simulink model "fig529a"  (Simulink 3.00)
settings: Solver=ode45  SolverMode=SingleTasking  StartTime=0.0  StopTime=2  RelTol=1e-3  AbsTol=1e-6
libraries: simulink3 x2

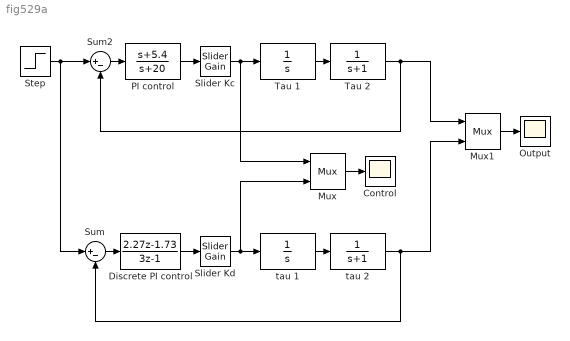
== system fig529a ==
  Control : Scope
      settings: TickLabels=on  TimeRange=auto  YMin=0  YMax=2.75  SaveName=ucd  DataFormat=Matrix
  Discrete PI control : DiscreteTransferFcn  Numerator=[2.27 -1.73]  Denominator=[3 -1]  SampleTime=.05
  Mux : Mux  Inputs=2
      settings: DisplayOption=none
  Mux1 : Mux  Inputs=2
      settings: DisplayOption=none
  Output : Scope
      settings: TickLabels=on  TimeRange=auto  YMin=-5  YMax=5  SaveName=ycd  DataFormat=Matrix
  PI control : TransferFcn  Numerator=[1 5.4]  Denominator=[1 20]
  Slider Kc : simulink3/Math/Slider Gain  low=0  gain=127  high=200
  Slider Kd : simulink3/Math/Slider Gain  low=0  gain=127  high=200
  Step : Step  Time=.1  Before=0  After=1  SampleTime=.001
  Sum : Sum  Inputs=|+-  SaturateOnIntegerOverflow=off
  Sum2 : Sum  Inputs=|+-  SaturateOnIntegerOverflow=off
  Tau 1 : TransferFcn  Numerator=[1]  Denominator=[1 0]
  Tau 2 : TransferFcn  Numerator=[1]  Denominator=[1 1]
  tau 1 : TransferFcn  Numerator=[1]  Denominator=[1 0]
  tau 2 : TransferFcn  Numerator=[1]  Denominator=[1 1]
  wires:
  PI control/1 -> Slider Kc/1
  Sum2/1 -> PI control/1
  Tau 1/1 -> Tau 2/1
  Discrete PI control/1 -> Slider Kd/1
  tau 1/1 -> tau 2/1
  Step/1 -> Sum2/1, Sum/1
  Slider Kc/1 -> Tau 1/1, Mux/1
  Mux/1 -> Control/1
  Tau 2/1 -> Mux1/1, Sum2/2
  Mux1/1 -> Output/1
  Sum/1 -> Discrete PI control/1
  Slider Kd/1 -> tau 1/1, Mux/2
  tau 2/1 -> Mux1/2, Sum/2
